simulink model "sin_model"  (R2021a)
settings: Solver=VariableStepAuto  StartTime=0.0  StopTime=10.0  RelTol=1e-3
PreLoadFcn:
  | sin_params
values from neighbouring files (symbols this model uses):
  A = 20    [sin_params.m]
  w = pi / 4    (= 0.785398163397)    [sin_params.m]
settings Model: Creator=User  LastModifiedBy=ampil

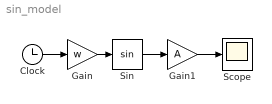
== system sin_model ==
  Clock : Clock
  Gain : Gain  Gain=w
  Gain1 : Gain  Gain=A
  Scope : Scope
  Sin : Trigonometry
  wires:
  Clock/1 -> Gain/1
  Gain/1 -> Sin/1
  Sin/1 -> Gain1/1
  Gain1/1 -> Scope/1
